simulink model "PTTransmCU"  (R2022b)
settings: Solver=ode45  StartTime=0.0  StopTime=inf  RelTol=1e-3  EnableMultiTasking=on
libraries: simulink x2, CarMaker4SL x1
(part 3 of 5)

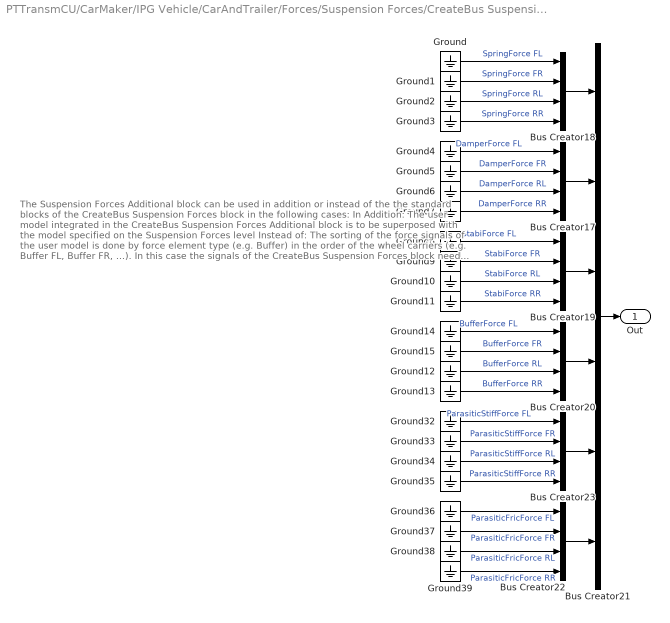
== system PTTransmCU/CarMaker/IPG Vehicle/CarAndTrailer/Forces/Suspension Forces/CreateBus Suspension Forces Additional ==
  note: The Suspension Forces Additional block can be used in addition or instead of the
      | the standard blocks of the CreateBus Suspension Forces block in the following cases:
      |
      | In Addition: The user model integrated in the CreateBus Suspension Forces Additional block is to be superposed with the model specified on the Suspension Forces level
      | Instead of: The sorting of the force signals of the user model is done by force element type (e.g. Buffer) in the order of the wheel carriers (e.g. Buffer FL, Buffer FR, ...). In this case the signals of the CreateBus Suspension Forces block need to be disabled e.g. by manually connecting them to ground signals.
      |
      | ATTENTION : The forces given in the CreateBus Suspension Forces Additional block are internally added to the forces of the Suspension Forces block. If this is not desired, make sure to include a force model only in one of the two levels.
  Bus Creator{17..20,22..23} (6 alike) : BusCreator  Inputs=4
  Bus Creator21 : BusCreator  Inputs=6
  Ground{,1..15,32..39} (24 alike) : Ground
  Out : Outport
  wires:
  Ground1/1 -> Bus Creator18/2  "SpringForce FR"
  Ground9/1 -> Bus Creator19/2  "StabiForce FR"
  Ground8/1 -> Bus Creator19/1  "StabiForce FL"
  Bus Creator22/1 -> Bus Creator21/6
  Bus Creator21/1 -> Out/1
  Ground/1 -> Bus Creator18/1  "SpringForce FL"
  Ground36/1 -> Bus Creator22/1  "ParasiticFricForce FL"
  Ground2/1 -> Bus Creator18/3  "SpringForce RL"
  Ground5/1 -> Bus Creator17/2  "DamperForce FR"
  Ground15/1 -> Bus Creator20/2  "BufferForce FR"
  Ground35/1 -> Bus Creator23/4  "ParasiticStiffForce RR"
  Bus Creator20/1 -> Bus Creator21/4
  Bus Creator17/1 -> Bus Creator21/2
  Ground37/1 -> Bus Creator22/2  "ParasiticFricForce FR"
  Ground4/1 -> Bus Creator17/1  "DamperForce FL"
  Ground33/1 -> Bus Creator23/2  "ParasiticStiffForce FR"
  Bus Creator23/1 -> Bus Creator21/5
  Ground11/1 -> Bus Creator19/4  "StabiForce RR"
  Ground10/1 -> Bus Creator19/3  "StabiForce RL"
  Ground6/1 -> Bus Creator17/3  "DamperForce RL"
  Bus Creator19/1 -> Bus Creator21/3
  Ground7/1 -> Bus Creator17/4  "DamperForce RR"
  Bus Creator18/1 -> Bus Creator21/1
  Ground34/1 -> Bus Creator23/3  "ParasiticStiffForce RL"
  Ground3/1 -> Bus Creator18/4  "SpringForce RR"
  Ground12/1 -> Bus Creator20/3  "BufferForce RL"
  Ground38/1 -> Bus Creator22/3  "ParasiticFricForce RL"
  Ground14/1 -> Bus Creator20/1  "BufferForce FL"
  Ground39/1 -> Bus Creator22/4  "ParasiticFricForce RR"
  Ground32/1 -> Bus Creator23/1  "ParasiticStiffForce FL"
  Ground13/1 -> Bus Creator20/4  "BufferForce RR"

== system PTTransmCU/CarMaker/IPG Vehicle/CarAndTrailer/Forces/Suspension Forces/CreateBus Suspension Forces CtrlOut ==
  note: <Your model here>
  In : Inport
  Bus Creator{,1..3,9} (5 alike) : BusCreator  Inputs=4
  Demux{,2..5} (5 alike) : Demux
  Out : Outport
  wires:
  Bus Creator3/1 -> Bus Creator9/4
  Demux2/4 -> Bus Creator/4  "FL BufferCtrlOut"
  Demux/4 -> Demux5/1  "RR"
  Bus Creator2/1 -> Bus Creator9/3
  Demux3/1 -> Bus Creator1/1  "FR SpringCtrlOut"
  Bus Creator/1 -> Bus Creator9/1
  Demux5/1 -> Bus Creator3/1  "RR SpringCtrlOut"
  Demux5/2 -> Bus Creator3/2  "RR DamperCtrlOut"
  Demux4/2 -> Bus Creator2/2  "RL DamperCtrlOut"
  Demux4/3 -> Bus Creator2/3  "RL StabiCtrlOut"
  Demux2/2 -> Bus Creator/2  "FL DamperCtrlOut"
  Demux/3 -> Demux4/1  "RL"
  Demux5/4 -> Bus Creator3/4  "RR BufferCtrlOut"
  In/1 -> Demux/1
  Demux2/1 -> Bus Creator/1  "FL SpringCtrlOut"
  Demux3/3 -> Bus Creator1/3  "FR StabiCtrlOut"
  Demux3/2 -> Bus Creator1/2  "FR DamperCtrlOut"
  Demux4/1 -> Bus Creator2/1  "RL SpringCtrlOut"
  Demux4/4 -> Bus Creator2/4  "RL BufferCtrlOut"
  Demux2/3 -> Bus Creator/3  "FL StabiCtrlOut"
  Bus Creator1/1 -> Bus Creator9/2
  Bus Creator9/1 -> Out/1
  Demux/1 -> Demux2/1  "FL"
  Demux/2 -> Demux3/1  "FR"
  Demux5/3 -> Bus Creator3/3  "RR StabiCtrlOut"
  Demux3/4 -> Bus Creator1/4  "FR BufferCtrlOut"

== system PTTransmCU/CarMaker/IPG Vehicle/CarAndTrailer/Forces/Suspension Forces/Damper CreateBus CtrlOutOpt ==
  note: <Your model here>
  In : Inport
  Bus Creator{,1..3,9} (5 alike) : BusCreator  Inputs=4
  Demux{,2..5} (5 alike) : Demux
  Out : Outport
  wires:
  Bus Creator/1 -> Bus Creator9/1
  Demux/4 -> Demux5/1  "RR"
  Bus Creator2/1 -> Bus Creator9/3
  Demux5/1 -> Bus Creator3/1  "RR CtrlOutOpt0"
  Bus Creator3/1 -> Bus Creator9/4
  Demux2/4 -> Bus Creator/4  "FL CtrlOutOpt3"
  Demux5/3 -> Bus Creator3/3  "RR CtrlOutOpt2"
  Demux4/3 -> Bus Creator2/3  "RL CtrlOutOpt2"
  Bus Creator1/1 -> Bus Creator9/2
  Demux4/2 -> Bus Creator2/2  "RL CtrlOutOpt1"
  Demux2/2 -> Bus Creator/2  "FL CtrlOutOpt1"
  Demux/2 -> Demux3/1  "FR"
  Demux3/4 -> Bus Creator1/4  "FR CtrlOutOpt3"
  Demux3/1 -> Bus Creator1/1  "FR CtrlOutOpt0"
  Demux4/4 -> Bus Creator2/4  "RL CtrlOutOpt3"
  Demux2/3 -> Bus Creator/3  "FL CtrlOutOpt2"
  Demux3/2 -> Bus Creator1/2  "FR CtrlOutOpt1"
  Demux2/1 -> Bus Creator/1  "FL CtrlOutOpt0"
  Demux3/3 -> Bus Creator1/3  "FR CtrlOutOpt2"
  In/1 -> Demux/1
  Demux5/4 -> Bus Creator3/4  "RR CtrlOutOpt3"
  Demux/3 -> Demux4/1  "RL"
  Bus Creator9/1 -> Out/1
  Demux5/2 -> Bus Creator3/2  "RR CtrlOutOpt1"
  Demux4/1 -> Bus Creator2/1  "RL CtrlOutOpt0"
  Demux/1 -> Demux2/1  "FL"

== system PTTransmCU/CarMaker/IPG Vehicle/CarAndTrailer/Forces/Suspension Forces/FrcSystem CreateBus CtrlOutOpt ==
  note: <Your model here>
  In : Inport
  Bus Creator9 : BusCreator  Inputs=64
  Demux : Demux  Outputs=64
  Out : Outport
  wires:
  In/1 -> Demux/1
  Bus Creator9/1 -> Out/1
  Demux/64 -> Bus Creator9/64  "CtrlOutOpt63"
  Demux/1 -> Bus Creator9/1  "CtrlOutOpt0"
  Demux/2 -> Bus Creator9/2  "CtrlOutOpt1"
  Demux/3 -> Bus Creator9/3  "CtrlOutOpt2"
  Demux/4 -> Bus Creator9/4  "CtrlOutOpt3"
  Demux/5 -> Bus Creator9/5  "CtrlOutOpt4"
  Demux/6 -> Bus Creator9/6  "CtrlOutOpt5"
  Demux/7 -> Bus Creator9/7  "CtrlOutOpt6"
  Demux/8 -> Bus Creator9/8  "CtrlOutOpt7"
  Demux/9 -> Bus Creator9/9  "CtrlOutOpt8"
  Demux/10 -> Bus Creator9/10  "CtrlOutOpt9"
  Demux/11 -> Bus Creator9/11  "CtrlOutOpt10"
  Demux/12 -> Bus Creator9/12  "CtrlOutOpt11"
  Demux/13 -> Bus Creator9/13  "CtrlOutOpt12"
  Demux/14 -> Bus Creator9/14  "CtrlOutOpt13"
  Demux/15 -> Bus Creator9/15  "CtrlOutOpt14"
  Demux/16 -> Bus Creator9/16  "CtrlOutOpt15"
  Demux/17 -> Bus Creator9/17  "CtrlOutOpt16"
  Demux/18 -> Bus Creator9/18  "CtrlOutOpt17"
  Demux/19 -> Bus Creator9/19  "CtrlOutOpt18"
  Demux/20 -> Bus Creator9/20  "CtrlOutOpt19"
  Demux/21 -> Bus Creator9/21  "CtrlOutOpt20"
  Demux/22 -> Bus Creator9/22  "CtrlOutOpt21"
  Demux/23 -> Bus Creator9/23  "CtrlOutOpt22"
  Demux/24 -> Bus Creator9/24  "CtrlOutOpt23"
  Demux/25 -> Bus Creator9/25  "CtrlOutOpt24"
  Demux/26 -> Bus Creator9/26  "CtrlOutOpt25"
  Demux/27 -> Bus Creator9/27  "CtrlOutOpt26"
  Demux/28 -> Bus Creator9/28  "CtrlOutOpt27"
  Demux/29 -> Bus Creator9/29  "CtrlOutOpt28"
  Demux/30 -> Bus Creator9/30  "CtrlOutOpt29"
  Demux/31 -> Bus Creator9/31  "CtrlOutOpt30"
  Demux/32 -> Bus Creator9/32  "CtrlOutOpt31"
  Demux/33 -> Bus Creator9/33  "CtrlOutOpt32"
  Demux/34 -> Bus Creator9/34  "CtrlOutOpt33"
  Demux/35 -> Bus Creator9/35  "CtrlOutOpt34"
  Demux/36 -> Bus Creator9/36  "CtrlOutOpt35"
  Demux/37 -> Bus Creator9/37  "CtrlOutOpt36"
  Demux/38 -> Bus Creator9/38  "CtrlOutOpt37"
  Demux/39 -> Bus Creator9/39  "CtrlOutOpt38"
  Demux/40 -> Bus Creator9/40  "CtrlOutOpt39"
  Demux/41 -> Bus Creator9/41  "CtrlOutOpt40"
  Demux/42 -> Bus Creator9/42  "CtrlOutOpt41"
  Demux/43 -> Bus Creator9/43  "CtrlOutOpt42"
  Demux/44 -> Bus Creator9/44  "CtrlOutOpt43"
  Demux/45 -> Bus Creator9/45  "CtrlOutOpt44"
  Demux/46 -> Bus Creator9/46  "CtrlOutOpt45"
  Demux/47 -> Bus Creator9/47  "CtrlOutOpt46"
  Demux/48 -> Bus Creator9/48  "CtrlOutOpt47"
  Demux/49 -> Bus Creator9/49  "CtrlOutOpt48"
  Demux/50 -> Bus Creator9/50  "CtrlOutOpt49"
  Demux/51 -> Bus Creator9/51  "CtrlOutOpt50"
  Demux/52 -> Bus Creator9/52  "CtrlOutOpt51"
  Demux/53 -> Bus Creator9/53  "CtrlOutOpt52"
  Demux/54 -> Bus Creator9/54  "CtrlOutOpt53"
  Demux/55 -> Bus Creator9/55  "CtrlOutOpt54"
  Demux/56 -> Bus Creator9/56  "CtrlOutOpt55"
  Demux/57 -> Bus Creator9/57  "CtrlOutOpt56"
  Demux/58 -> Bus Creator9/58  "CtrlOutOpt57"
  Demux/59 -> Bus Creator9/59  "CtrlOutOpt58"
  Demux/60 -> Bus Creator9/60  "CtrlOutOpt59"
  Demux/61 -> Bus Creator9/61  "CtrlOutOpt60"
  Demux/62 -> Bus Creator9/62  "CtrlOutOpt61"
  Demux/63 -> Bus Creator9/63  "CtrlOutOpt62"

== system PTTransmCU/CarMaker/IPG Vehicle/CarAndTrailer/Forces/Suspension Forces/Spring CreateBus CtrlOutOpt ==
  note: <Your model here>
  In : Inport
  Bus Creator{,1..3,9} (5 alike) : BusCreator  Inputs=4
  Demux{,2..5} (5 alike) : Demux
  Out : Outport
  wires:
  Bus Creator/1 -> Bus Creator9/1
  Demux/4 -> Demux5/1  "RR"
  Bus Creator2/1 -> Bus Creator9/3
  Demux5/1 -> Bus Creator3/1  "RR CtrlOutOpt0"
  Bus Creator3/1 -> Bus Creator9/4
  Demux2/4 -> Bus Creator/4  "FL CtrlOutOpt3"
  Demux5/3 -> Bus Creator3/3  "RR CtrlOutOpt2"
  Demux4/3 -> Bus Creator2/3  "RL CtrlOutOpt2"
  Bus Creator1/1 -> Bus Creator9/2
  Demux4/2 -> Bus Creator2/2  "RL CtrlOutOpt1"
  Demux2/2 -> Bus Creator/2  "FL CtrlOutOpt1"
  Demux/2 -> Demux3/1  "FR"
  Demux3/4 -> Bus Creator1/4  "FR CtrlOutOpt3"
  Demux3/1 -> Bus Creator1/1  "FR CtrlOutOpt0"
  Demux4/4 -> Bus Creator2/4  "RL CtrlOutOpt3"
  Demux2/3 -> Bus Creator/3  "FL CtrlOutOpt2"
  Demux3/2 -> Bus Creator1/2  "FR CtrlOutOpt1"
  Demux2/1 -> Bus Creator/1  "FL CtrlOutOpt0"
  Demux3/3 -> Bus Creator1/3  "FR CtrlOutOpt2"
  In/1 -> Demux/1
  Demux5/4 -> Bus Creator3/4  "RR CtrlOutOpt3"
  Demux/3 -> Demux4/1  "RL"
  Bus Creator9/1 -> Out/1
  Demux5/2 -> Bus Creator3/2  "RR CtrlOutOpt1"
  Demux4/1 -> Bus Creator2/1  "RL CtrlOutOpt0"
  Demux/1 -> Demux2/1  "FL"

== system PTTransmCU/CarMaker/IPG Vehicle/CarAndTrailer/Forces/Suspension Forces/Stabi CreateBus CtrlOutOpt ==
  note: <Your model here>
  In : Inport
  Bus Creator{,1..3,9} (5 alike) : BusCreator  Inputs=4
  Demux{,2..5} (5 alike) : Demux
  Out : Outport
  wires:
  Bus Creator/1 -> Bus Creator9/1
  Demux/4 -> Demux5/1  "RR"
  Bus Creator2/1 -> Bus Creator9/3
  Demux5/1 -> Bus Creator3/1  "RR CtrlOutOpt0"
  Bus Creator3/1 -> Bus Creator9/4
  Demux2/4 -> Bus Creator/4  "FL CtrlOutOpt3"
  Demux5/3 -> Bus Creator3/3  "RR CtrlOutOpt2"
  Demux4/3 -> Bus Creator2/3  "RL CtrlOutOpt2"
  Bus Creator1/1 -> Bus Creator9/2
  Demux4/2 -> Bus Creator2/2  "RL CtrlOutOpt1"
  Demux2/2 -> Bus Creator/2  "FL CtrlOutOpt1"
  Demux/2 -> Demux3/1  "FR"
  Demux3/4 -> Bus Creator1/4  "FR CtrlOutOpt3"
  Demux3/1 -> Bus Creator1/1  "FR CtrlOutOpt0"
  Demux4/4 -> Bus Creator2/4  "RL CtrlOutOpt3"
  Demux2/3 -> Bus Creator/3  "FL CtrlOutOpt2"
  Demux3/2 -> Bus Creator1/2  "FR CtrlOutOpt1"
  Demux2/1 -> Bus Creator/1  "FL CtrlOutOpt0"
  Demux3/3 -> Bus Creator1/3  "FR CtrlOutOpt2"
  In/1 -> Demux/1
  Demux5/4 -> Bus Creator3/4  "RR CtrlOutOpt3"
  Demux/3 -> Demux4/1  "RL"
  Bus Creator9/1 -> Out/1
  Demux5/2 -> Bus Creator3/2  "RR CtrlOutOpt1"
  Demux4/1 -> Bus Creator2/1  "RL CtrlOutOpt0"
  Demux/1 -> Demux2/1  "FL"

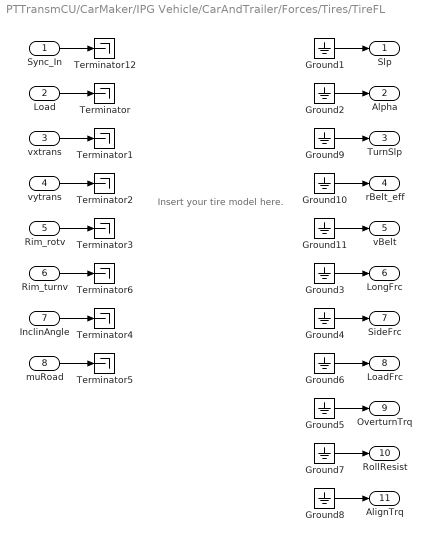
== system PTTransmCU/CarMaker/IPG Vehicle/CarAndTrailer/Forces/Tires/TireFL ==
  note: Insert your tire model here.
  Sync_In : Inport
  Load : Inport  Port=2
  vxtrans : Inport  Port=3
  vytrans : Inport  Port=4
  Rim_rotv : Inport  Port=5
  Rim_turnv : Inport  Port=6
  InclinAngle : Inport  Port=7
  muRoad : Inport  Port=8
  Ground{1..11} (11 alike) : Ground
  Terminator{,1..6,12} (8 alike) : Terminator
  Slp : Outport  VectorParamsAs1DForOutWhenUnconnected=off
  Alpha : Outport  Port=2  VectorParamsAs1DForOutWhenUnconnected=off
  TurnSlp : Outport  Port=3  VectorParamsAs1DForOutWhenUnconnected=off
  rBelt_eff : Outport  Port=4  VectorParamsAs1DForOutWhenUnconnected=off
  vBelt : Outport  Port=5  VectorParamsAs1DForOutWhenUnconnected=off
  LongFrc : Outport  Port=6  VectorParamsAs1DForOutWhenUnconnected=off
  SideFrc : Outport  Port=7  VectorParamsAs1DForOutWhenUnconnected=off
  LoadFrc : Outport  Port=8  VectorParamsAs1DForOutWhenUnconnected=off
  OverturnTrq : Outport  Port=9  VectorParamsAs1DForOutWhenUnconnected=off
  RollResist : Outport  Port=10  VectorParamsAs1DForOutWhenUnconnected=off
  AlignTrq : Outport  Port=11  VectorParamsAs1DForOutWhenUnconnected=off
  wires:
  Ground11/1 -> vBelt/1
  Ground10/1 -> rBelt_eff/1
  Ground9/1 -> TurnSlp/1
  Rim_turnv/1 -> Terminator6/1
  Sync_In/1 -> Terminator12/1
  Ground2/1 -> Alpha/1
  Ground3/1 -> LongFrc/1
  Ground4/1 -> SideFrc/1
  Ground5/1 -> OverturnTrq/1
  vxtrans/1 -> Terminator1/1
  vytrans/1 -> Terminator2/1
  Rim_rotv/1 -> Terminator3/1
  InclinAngle/1 -> Terminator4/1
  muRoad/1 -> Terminator5/1
  Load/1 -> Terminator/1
  Ground1/1 -> Slp/1
  Ground6/1 -> LoadFrc/1
  Ground7/1 -> RollResist/1
  Ground8/1 -> AlignTrq/1

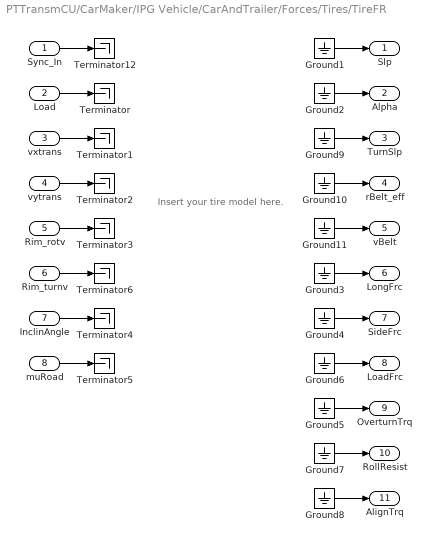
== system PTTransmCU/CarMaker/IPG Vehicle/CarAndTrailer/Forces/Tires/TireFR ==
  note: Insert your tire model here.
  Sync_In : Inport
  Load : Inport  Port=2
  vxtrans : Inport  Port=3
  vytrans : Inport  Port=4
  Rim_rotv : Inport  Port=5
  Rim_turnv : Inport  Port=6
  InclinAngle : Inport  Port=7
  muRoad : Inport  Port=8
  Ground{1..11} (11 alike) : Ground
  Terminator{,1..6,12} (8 alike) : Terminator
  Slp : Outport  VectorParamsAs1DForOutWhenUnconnected=off
  Alpha : Outport  Port=2  VectorParamsAs1DForOutWhenUnconnected=off
  TurnSlp : Outport  Port=3  VectorParamsAs1DForOutWhenUnconnected=off
  rBelt_eff : Outport  Port=4  VectorParamsAs1DForOutWhenUnconnected=off
  vBelt : Outport  Port=5  VectorParamsAs1DForOutWhenUnconnected=off
  LongFrc : Outport  Port=6  VectorParamsAs1DForOutWhenUnconnected=off
  SideFrc : Outport  Port=7  VectorParamsAs1DForOutWhenUnconnected=off
  LoadFrc : Outport  Port=8  VectorParamsAs1DForOutWhenUnconnected=off
  OverturnTrq : Outport  Port=9  VectorParamsAs1DForOutWhenUnconnected=off
  RollResist : Outport  Port=10  VectorParamsAs1DForOutWhenUnconnected=off
  AlignTrq : Outport  Port=11  VectorParamsAs1DForOutWhenUnconnected=off
  wires:
  Ground11/1 -> vBelt/1
  Ground10/1 -> rBelt_eff/1
  Ground9/1 -> TurnSlp/1
  Rim_turnv/1 -> Terminator6/1
  Sync_In/1 -> Terminator12/1
  Ground2/1 -> Alpha/1
  Ground3/1 -> LongFrc/1
  Ground4/1 -> SideFrc/1
  Ground5/1 -> OverturnTrq/1
  vxtrans/1 -> Terminator1/1
  vytrans/1 -> Terminator2/1
  Rim_rotv/1 -> Terminator3/1
  InclinAngle/1 -> Terminator4/1
  muRoad/1 -> Terminator5/1
  Load/1 -> Terminator/1
  Ground1/1 -> Slp/1
  Ground6/1 -> LoadFrc/1
  Ground7/1 -> RollResist/1
  Ground8/1 -> AlignTrq/1

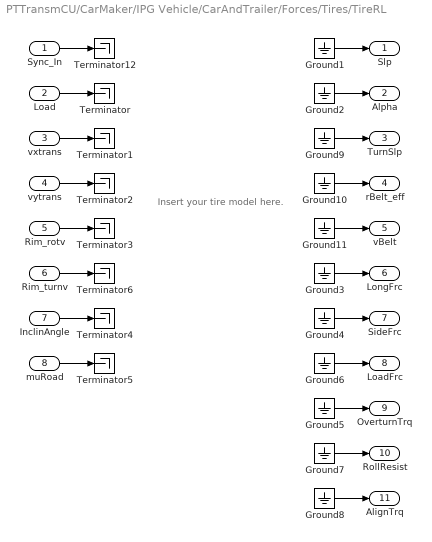
== system PTTransmCU/CarMaker/IPG Vehicle/CarAndTrailer/Forces/Tires/TireRL ==
  note: Insert your tire model here.
  Sync_In : Inport
  Load : Inport  Port=2
  vxtrans : Inport  Port=3
  vytrans : Inport  Port=4
  Rim_rotv : Inport  Port=5
  Rim_turnv : Inport  Port=6
  InclinAngle : Inport  Port=7
  muRoad : Inport  Port=8
  Ground{1..11} (11 alike) : Ground
  Terminator{,1..6,12} (8 alike) : Terminator
  Slp : Outport  VectorParamsAs1DForOutWhenUnconnected=off
  Alpha : Outport  Port=2  VectorParamsAs1DForOutWhenUnconnected=off
  TurnSlp : Outport  Port=3  VectorParamsAs1DForOutWhenUnconnected=off
  rBelt_eff : Outport  Port=4  VectorParamsAs1DForOutWhenUnconnected=off
  vBelt : Outport  Port=5  VectorParamsAs1DForOutWhenUnconnected=off
  LongFrc : Outport  Port=6  VectorParamsAs1DForOutWhenUnconnected=off
  SideFrc : Outport  Port=7  VectorParamsAs1DForOutWhenUnconnected=off
  LoadFrc : Outport  Port=8  VectorParamsAs1DForOutWhenUnconnected=off
  OverturnTrq : Outport  Port=9  VectorParamsAs1DForOutWhenUnconnected=off
  RollResist : Outport  Port=10  VectorParamsAs1DForOutWhenUnconnected=off
  AlignTrq : Outport  Port=11  VectorParamsAs1DForOutWhenUnconnected=off
  wires:
  Ground11/1 -> vBelt/1
  Ground10/1 -> rBelt_eff/1
  Ground9/1 -> TurnSlp/1
  Rim_turnv/1 -> Terminator6/1
  Sync_In/1 -> Terminator12/1
  Ground2/1 -> Alpha/1
  Ground3/1 -> LongFrc/1
  Ground4/1 -> SideFrc/1
  Ground5/1 -> OverturnTrq/1
  vxtrans/1 -> Terminator1/1
  vytrans/1 -> Terminator2/1
  Rim_rotv/1 -> Terminator3/1
  InclinAngle/1 -> Terminator4/1
  muRoad/1 -> Terminator5/1
  Load/1 -> Terminator/1
  Ground1/1 -> Slp/1
  Ground6/1 -> LoadFrc/1
  Ground7/1 -> RollResist/1
  Ground8/1 -> AlignTrq/1

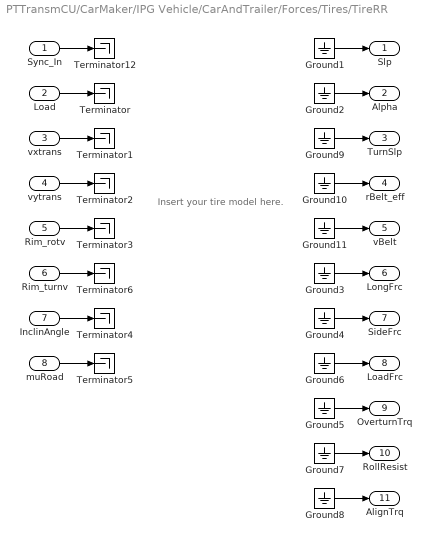
== system PTTransmCU/CarMaker/IPG Vehicle/CarAndTrailer/Forces/Tires/TireRR ==
  note: Insert your tire model here.
  Sync_In : Inport
  Load : Inport  Port=2
  vxtrans : Inport  Port=3
  vytrans : Inport  Port=4
  Rim_rotv : Inport  Port=5
  Rim_turnv : Inport  Port=6
  InclinAngle : Inport  Port=7
  muRoad : Inport  Port=8
  Ground{1..11} (11 alike) : Ground
  Terminator{,1..6,12} (8 alike) : Terminator
  Slp : Outport  VectorParamsAs1DForOutWhenUnconnected=off
  Alpha : Outport  Port=2  VectorParamsAs1DForOutWhenUnconnected=off
  TurnSlp : Outport  Port=3  VectorParamsAs1DForOutWhenUnconnected=off
  rBelt_eff : Outport  Port=4  VectorParamsAs1DForOutWhenUnconnected=off
  vBelt : Outport  Port=5  VectorParamsAs1DForOutWhenUnconnected=off
  LongFrc : Outport  Port=6  VectorParamsAs1DForOutWhenUnconnected=off
  SideFrc : Outport  Port=7  VectorParamsAs1DForOutWhenUnconnected=off
  LoadFrc : Outport  Port=8  VectorParamsAs1DForOutWhenUnconnected=off
  OverturnTrq : Outport  Port=9  VectorParamsAs1DForOutWhenUnconnected=off
  RollResist : Outport  Port=10  VectorParamsAs1DForOutWhenUnconnected=off
  AlignTrq : Outport  Port=11  VectorParamsAs1DForOutWhenUnconnected=off
  wires:
  Ground11/1 -> vBelt/1
  Ground10/1 -> rBelt_eff/1
  Ground9/1 -> TurnSlp/1
  Rim_turnv/1 -> Terminator6/1
  Sync_In/1 -> Terminator12/1
  Ground2/1 -> Alpha/1
  Ground3/1 -> LongFrc/1
  Ground4/1 -> SideFrc/1
  Ground5/1 -> OverturnTrq/1
  vxtrans/1 -> Terminator1/1
  vytrans/1 -> Terminator2/1
  Rim_rotv/1 -> Terminator3/1
  InclinAngle/1 -> Terminator4/1
  muRoad/1 -> Terminator5/1
  Load/1 -> Terminator/1
  Ground1/1 -> Slp/1
  Ground6/1 -> LoadFrc/1
  Ground7/1 -> RollResist/1
  Ground8/1 -> AlignTrq/1

== system PTTransmCU/CarMaker/IPG Vehicle/PowerTrain/TCU Example/PTTransmCU_In/CreateBus TCU ClutchIn0 ==
  In : Inport
  BusCreator : BusCreator  Inputs=7
  Demux : Demux  Outputs=7
      settings: DisplayOption=none
  Out : Outport  VectorParamsAs1DForOutWhenUnconnected=off
  wires:
  Demux/7 -> BusCreator/7  "TCU ClutchIn0 i_TrqIn2Out"
  Demux/6 -> BusCreator/6  "TCU ClutchIn0 Trq_out_trg"
  Demux/5 -> BusCreator/5  "TCU ClutchIn0 Trq_out"
  Demux/4 -> BusCreator/4  "TCU ClutchIn0 Trq_in"
  Demux/3 -> BusCreator/3  "TCU ClutchIn0 rotv_out_trg"
  Demux/2 -> BusCreator/2  "TCU ClutchIn0 rotv_out"
  Demux/1 -> BusCreator/1  "TCU ClutchIn0 rotv_in"
  BusCreator/1 -> Out/1
  In/1 -> Demux/1

== system PTTransmCU/CarMaker/IPG Vehicle/PowerTrain/TCU Example/PTTransmCU_In/CreateBus TCU ClutchIn1 ==
  In : Inport
  BusCreator : BusCreator  Inputs=7
  Demux : Demux  Outputs=7
      settings: DisplayOption=none
  Out : Outport  VectorParamsAs1DForOutWhenUnconnected=off
  wires:
  Demux/7 -> BusCreator/7  "TCU ClutchIn1 i_TrqIn2Out"
  Demux/6 -> BusCreator/6  "TCU ClutchIn1 Trq_out_trg"
  Demux/5 -> BusCreator/5  "TCU ClutchIn1 Trq_out"
  Demux/4 -> BusCreator/4  "TCU ClutchIn1 Trq_in"
  Demux/3 -> BusCreator/3  "TCU ClutchIn1 rotv_out_trg"
  Demux/2 -> BusCreator/2  "TCU ClutchIn1 rotv_out"
  Demux/1 -> BusCreator/1  "TCU ClutchIn1 rotv_in"
  BusCreator/1 -> Out/1
  In/1 -> Demux/1

== system PTTransmCU/CarMaker/IPG Vehicle/PowerTrain/TCU Example/PTTransmCU_In/CreateBus TCU ClutchIn10 ==
  In : Inport
  BusCreator : BusCreator  Inputs=7
  Demux : Demux  Outputs=7
      settings: DisplayOption=none
  Out : Outport  VectorParamsAs1DForOutWhenUnconnected=off
  wires:
  Demux/7 -> BusCreator/7  "TCU ClutchIn10 i_TrqIn2Out"
  Demux/6 -> BusCreator/6  "TCU ClutchIn10 Trq_out_trg"
  Demux/5 -> BusCreator/5  "TCU ClutchIn10 Trq_out"
  Demux/4 -> BusCreator/4  "TCU ClutchIn10 Trq_in"
  Demux/3 -> BusCreator/3  "TCU ClutchIn10 rotv_out_trg"
  Demux/2 -> BusCreator/2  "TCU ClutchIn10 rotv_out"
  Demux/1 -> BusCreator/1  "TCU ClutchIn10 rotv_in"
  BusCreator/1 -> Out/1
  In/1 -> Demux/1

== system PTTransmCU/CarMaker/IPG Vehicle/PowerTrain/TCU Example/PTTransmCU_In/CreateBus TCU ClutchIn11 ==
  In : Inport
  BusCreator : BusCreator  Inputs=7
  Demux : Demux  Outputs=7
      settings: DisplayOption=none
  Out : Outport  VectorParamsAs1DForOutWhenUnconnected=off
  wires:
  Demux/7 -> BusCreator/7  "TCU ClutchIn10 i_TrqIn2Out"
  Demux/6 -> BusCreator/6  "TCU ClutchIn10 Trq_out_trg"
  Demux/5 -> BusCreator/5  "TCU ClutchIn10 Trq_out"
  Demux/4 -> BusCreator/4  "TCU ClutchIn10 Trq_in"
  Demux/3 -> BusCreator/3  "TCU ClutchIn10 rotv_out_trg"
  Demux/2 -> BusCreator/2  "TCU ClutchIn10 rotv_out"
  Demux/1 -> BusCreator/1  "TCU ClutchIn10 rotv_in"
  BusCreator/1 -> Out/1
  In/1 -> Demux/1

== system PTTransmCU/CarMaker/IPG Vehicle/PowerTrain/TCU Example/PTTransmCU_In/CreateBus TCU ClutchIn2 ==
  In : Inport
  BusCreator : BusCreator  Inputs=7
  Demux : Demux  Outputs=7
      settings: DisplayOption=none
  Out : Outport  VectorParamsAs1DForOutWhenUnconnected=off
  wires:
  Demux/7 -> BusCreator/7  "TCU ClutchIn2 i_TrqIn2Out"
  Demux/6 -> BusCreator/6  "TCU ClutchIn2 Trq_out_trg"
  Demux/5 -> BusCreator/5  "TCU ClutchIn2 Trq_out"
  Demux/4 -> BusCreator/4  "TCU ClutchIn2 Trq_in"
  Demux/3 -> BusCreator/3  "TCU ClutchIn2 rotv_out_trg"
  Demux/2 -> BusCreator/2  "TCU ClutchIn2 rotv_out"
  Demux/1 -> BusCreator/1  "TCU ClutchIn2 rotv_in"
  BusCreator/1 -> Out/1
  In/1 -> Demux/1

== system PTTransmCU/CarMaker/IPG Vehicle/PowerTrain/TCU Example/PTTransmCU_In/CreateBus TCU ClutchIn3 ==
  In : Inport
  BusCreator : BusCreator  Inputs=7
  Demux : Demux  Outputs=7
      settings: DisplayOption=none
  Out : Outport  VectorParamsAs1DForOutWhenUnconnected=off
  wires:
  Demux/7 -> BusCreator/7  "TCU ClutchIn3 i_TrqIn2Out"
  Demux/6 -> BusCreator/6  "TCU ClutchIn3 Trq_out_trg"
  Demux/5 -> BusCreator/5  "TCU ClutchIn3 Trq_out"
  Demux/4 -> BusCreator/4  "TCU ClutchIn3 Trq_in"
  Demux/3 -> BusCreator/3  "TCU ClutchIn3 rotv_out_trg"
  Demux/2 -> BusCreator/2  "TCU ClutchIn3 rotv_out"
  Demux/1 -> BusCreator/1  "TCU ClutchIn3 rotv_in"
  BusCreator/1 -> Out/1
  In/1 -> Demux/1

== system PTTransmCU/CarMaker/IPG Vehicle/PowerTrain/TCU Example/PTTransmCU_In/CreateBus TCU ClutchIn4 ==
  In : Inport
  BusCreator : BusCreator  Inputs=7
  Demux : Demux  Outputs=7
      settings: DisplayOption=none
  Out : Outport  VectorParamsAs1DForOutWhenUnconnected=off
  wires:
  Demux/7 -> BusCreator/7  "TCU ClutchIn4 i_TrqIn2Out"
  Demux/6 -> BusCreator/6  "TCU ClutchIn4 Trq_out_trg"
  Demux/5 -> BusCreator/5  "TCU ClutchIn4 Trq_out"
  Demux/4 -> BusCreator/4  "TCU ClutchIn4 Trq_in"
  Demux/3 -> BusCreator/3  "TCU ClutchIn4 rotv_out_trg"
  Demux/2 -> BusCreator/2  "TCU ClutchIn4 rotv_out"
  Demux/1 -> BusCreator/1  "TCU ClutchIn4 rotv_in"
  BusCreator/1 -> Out/1
  In/1 -> Demux/1

== system PTTransmCU/CarMaker/IPG Vehicle/PowerTrain/TCU Example/PTTransmCU_In/CreateBus TCU ClutchIn5 ==
  In : Inport
  BusCreator : BusCreator  Inputs=7
  Demux : Demux  Outputs=7
      settings: DisplayOption=none
  Out : Outport  VectorParamsAs1DForOutWhenUnconnected=off
  wires:
  Demux/7 -> BusCreator/7  "TCU ClutchIn5 i_TrqIn2Out"
  Demux/6 -> BusCreator/6  "TCU ClutchIn5 Trq_out_trg"
  Demux/5 -> BusCreator/5  "TCU ClutchIn5 Trq_out"
  Demux/4 -> BusCreator/4  "TCU ClutchIn5 Trq_in"
  Demux/3 -> BusCreator/3  "TCU ClutchIn5 rotv_out_trg"
  Demux/2 -> BusCreator/2  "TCU ClutchIn5 rotv_out"
  Demux/1 -> BusCreator/1  "TCU ClutchIn5 rotv_in"
  BusCreator/1 -> Out/1
  In/1 -> Demux/1

== system PTTransmCU/CarMaker/IPG Vehicle/PowerTrain/TCU Example/PTTransmCU_In/CreateBus TCU ClutchIn6 ==
  In : Inport
  BusCreator : BusCreator  Inputs=7
  Demux : Demux  Outputs=7
      settings: DisplayOption=none
  Out : Outport  VectorParamsAs1DForOutWhenUnconnected=off
  wires:
  Demux/7 -> BusCreator/7  "TCU ClutchIn6 i_TrqIn2Out"
  Demux/6 -> BusCreator/6  "TCU ClutchIn6 Trq_out_trg"
  Demux/5 -> BusCreator/5  "TCU ClutchIn6 Trq_out"
  Demux/4 -> BusCreator/4  "TCU ClutchIn6 Trq_in"
  Demux/3 -> BusCreator/3  "TCU ClutchIn6 rotv_out_trg"
  Demux/2 -> BusCreator/2  "TCU ClutchIn6 rotv_out"
  Demux/1 -> BusCreator/1  "TCU ClutchIn6 rotv_in"
  BusCreator/1 -> Out/1
  In/1 -> Demux/1

== system PTTransmCU/CarMaker/IPG Vehicle/PowerTrain/TCU Example/PTTransmCU_In/CreateBus TCU ClutchIn7 ==
  In : Inport
  BusCreator : BusCreator  Inputs=7
  Demux : Demux  Outputs=7
      settings: DisplayOption=none
  Out : Outport  VectorParamsAs1DForOutWhenUnconnected=off
  wires:
  Demux/7 -> BusCreator/7  "TCU ClutchIn7 i_TrqIn2Out"
  Demux/6 -> BusCreator/6  "TCU ClutchIn7 Trq_out_trg"
  Demux/5 -> BusCreator/5  "TCU ClutchIn7 Trq_out"
  Demux/4 -> BusCreator/4  "TCU ClutchIn7 Trq_in"
  Demux/3 -> BusCreator/3  "TCU ClutchIn7 rotv_out_trg"
  Demux/2 -> BusCreator/2  "TCU ClutchIn7 rotv_out"
  Demux/1 -> BusCreator/1  "TCU ClutchIn7 rotv_in"
  BusCreator/1 -> Out/1
  In/1 -> Demux/1

== system PTTransmCU/CarMaker/IPG Vehicle/PowerTrain/TCU Example/PTTransmCU_In/CreateBus TCU ClutchIn8 ==
  In : Inport
  BusCreator : BusCreator  Inputs=7
  Demux : Demux  Outputs=7
      settings: DisplayOption=none
  Out : Outport  VectorParamsAs1DForOutWhenUnconnected=off
  wires:
  Demux/7 -> BusCreator/7  "TCU ClutchIn8 i_TrqIn2Out"
  Demux/6 -> BusCreator/6  "TCU ClutchIn8 Trq_out_trg"
  Demux/5 -> BusCreator/5  "TCU ClutchIn8 Trq_out"
  Demux/4 -> BusCreator/4  "TCU ClutchIn8 Trq_in"
  Demux/3 -> BusCreator/3  "TCU ClutchIn8 rotv_out_trg"
  Demux/2 -> BusCreator/2  "TCU ClutchIn8 rotv_out"
  Demux/1 -> BusCreator/1  "TCU ClutchIn8 rotv_in"
  BusCreator/1 -> Out/1
  In/1 -> Demux/1

== system PTTransmCU/CarMaker/IPG Vehicle/PowerTrain/TCU Example/PTTransmCU_In/CreateBus TCU ClutchIn9 ==
  In : Inport
  BusCreator : BusCreator  Inputs=7
  Demux : Demux  Outputs=7
      settings: DisplayOption=none
  Out : Outport  VectorParamsAs1DForOutWhenUnconnected=off
  wires:
  Demux/7 -> BusCreator/7  "TCU ClutchIn9 i_TrqIn2Out"
  Demux/6 -> BusCreator/6  "TCU ClutchIn9 Trq_out_trg"
  Demux/5 -> BusCreator/5  "TCU ClutchIn9 Trq_out"
  Demux/4 -> BusCreator/4  "TCU ClutchIn9 Trq_in"
  Demux/3 -> BusCreator/3  "TCU ClutchIn9 rotv_out_trg"
  Demux/2 -> BusCreator/2  "TCU ClutchIn9 rotv_out"
  Demux/1 -> BusCreator/1  "TCU ClutchIn9 rotv_in"
  BusCreator/1 -> Out/1
  In/1 -> Demux/1

== system PTTransmCU/CarMaker/IPG Vehicle/PowerTrain/TCU Example/PTTransmCU_In/CreateBus TCU ClutchOut0 ==
  In : Inport
  BusCreator : BusCreator  Inputs=1
  Demux : Demux  Outputs=1
      settings: DisplayOption=none
  Out : Outport  VectorParamsAs1DForOutWhenUnconnected=off
  wires:
  Demux/1 -> BusCreator/1  "TCU ClutchOut0 Pos"
  BusCreator/1 -> Out/1
  In/1 -> Demux/1

== system PTTransmCU/CarMaker/IPG Vehicle/PowerTrain/TCU Example/PTTransmCU_In/CreateBus TCU ClutchOut1 ==
  In : Inport
  BusCreator : BusCreator  Inputs=1
  Demux : Demux  Outputs=1
      settings: DisplayOption=none
  Out : Outport  VectorParamsAs1DForOutWhenUnconnected=off
  wires:
  Demux/1 -> BusCreator/1  "TCU ClutchOut1 Pos"
  BusCreator/1 -> Out/1
  In/1 -> Demux/1

== system PTTransmCU/CarMaker/IPG Vehicle/PowerTrain/TCU Example/PTTransmCU_In/CreateBus TCU ClutchOut10 ==
  In : Inport
  BusCreator : BusCreator  Inputs=1
  Demux : Demux  Outputs=1
      settings: DisplayOption=none
  Out : Outport  VectorParamsAs1DForOutWhenUnconnected=off
  wires:
  Demux/1 -> BusCreator/1  "TCU ClutchOut10 Pos"
  BusCreator/1 -> Out/1
  In/1 -> Demux/1

== system PTTransmCU/CarMaker/IPG Vehicle/PowerTrain/TCU Example/PTTransmCU_In/CreateBus TCU ClutchOut11 ==
  In : Inport
  BusCreator : BusCreator  Inputs=1
  Demux : Demux  Outputs=1
      settings: DisplayOption=none
  Out : Outport  VectorParamsAs1DForOutWhenUnconnected=off
  wires:
  Demux/1 -> BusCreator/1  "TCU ClutchOut11 Pos"
  BusCreator/1 -> Out/1
  In/1 -> Demux/1

== system PTTransmCU/CarMaker/IPG Vehicle/PowerTrain/TCU Example/PTTransmCU_In/CreateBus TCU ClutchOut2 ==
  In : Inport
  BusCreator : BusCreator  Inputs=1
  Demux : Demux  Outputs=1
      settings: DisplayOption=none
  Out : Outport  VectorParamsAs1DForOutWhenUnconnected=off
  wires:
  Demux/1 -> BusCreator/1  "TCU ClutchOut2 Pos"
  BusCreator/1 -> Out/1
  In/1 -> Demux/1

== system PTTransmCU/CarMaker/IPG Vehicle/PowerTrain/TCU Example/PTTransmCU_In/CreateBus TCU ClutchOut3 ==
  In : Inport
  BusCreator : BusCreator  Inputs=1
  Demux : Demux  Outputs=1
      settings: DisplayOption=none
  Out : Outport  VectorParamsAs1DForOutWhenUnconnected=off
  wires:
  Demux/1 -> BusCreator/1  "TCU ClutchOut3 Pos"
  BusCreator/1 -> Out/1
  In/1 -> Demux/1

== system PTTransmCU/CarMaker/IPG Vehicle/PowerTrain/TCU Example/PTTransmCU_In/CreateBus TCU ClutchOut4 ==
  In : Inport
  BusCreator : BusCreator  Inputs=1
  Demux : Demux  Outputs=1
      settings: DisplayOption=none
  Out : Outport  VectorParamsAs1DForOutWhenUnconnected=off
  wires:
  Demux/1 -> BusCreator/1  "TCU ClutchOut4 Pos"
  BusCreator/1 -> Out/1
  In/1 -> Demux/1

== system PTTransmCU/CarMaker/IPG Vehicle/PowerTrain/TCU Example/PTTransmCU_In/CreateBus TCU ClutchOut5 ==
  In : Inport
  BusCreator : BusCreator  Inputs=1
  Demux : Demux  Outputs=1
      settings: DisplayOption=none
  Out : Outport  VectorParamsAs1DForOutWhenUnconnected=off
  wires:
  Demux/1 -> BusCreator/1  "TCU ClutchOut5 Pos"
  BusCreator/1 -> Out/1
  In/1 -> Demux/1

== system PTTransmCU/CarMaker/IPG Vehicle/PowerTrain/TCU Example/PTTransmCU_In/CreateBus TCU ClutchOut6 ==
  In : Inport
  BusCreator : BusCreator  Inputs=1
  Demux : Demux  Outputs=1
      settings: DisplayOption=none
  Out : Outport  VectorParamsAs1DForOutWhenUnconnected=off
  wires:
  Demux/1 -> BusCreator/1  "TCU ClutchOut6 Pos"
  BusCreator/1 -> Out/1
  In/1 -> Demux/1

== system PTTransmCU/CarMaker/IPG Vehicle/PowerTrain/TCU Example/PTTransmCU_In/CreateBus TCU ClutchOut7 ==
  In : Inport
  BusCreator : BusCreator  Inputs=1
  Demux : Demux  Outputs=1
      settings: DisplayOption=none
  Out : Outport  VectorParamsAs1DForOutWhenUnconnected=off
  wires:
  Demux/1 -> BusCreator/1  "TCU ClutchOut7 Pos"
  BusCreator/1 -> Out/1
  In/1 -> Demux/1

== system PTTransmCU/CarMaker/IPG Vehicle/PowerTrain/TCU Example/PTTransmCU_In/CreateBus TCU ClutchOut8 ==
  In : Inport
  BusCreator : BusCreator  Inputs=1
  Demux : Demux  Outputs=1
      settings: DisplayOption=none
  Out : Outport  VectorParamsAs1DForOutWhenUnconnected=off
  wires:
  Demux/1 -> BusCreator/1  "TCU ClutchOut8 Pos"
  BusCreator/1 -> Out/1
  In/1 -> Demux/1

== system PTTransmCU/CarMaker/IPG Vehicle/PowerTrain/TCU Example/PTTransmCU_In/CreateBus TCU ClutchOut9 ==
  In : Inport
  BusCreator : BusCreator  Inputs=1
  Demux : Demux  Outputs=1
      settings: DisplayOption=none
  Out : Outport  VectorParamsAs1DForOutWhenUnconnected=off
  wires:
  Demux/1 -> BusCreator/1  "TCU ClutchOut9 Pos"
  BusCreator/1 -> Out/1
  In/1 -> Demux/1

== system PTTransmCU/CarMaker/IPG Vehicle/PowerTrain/TCU Example/PTTransmCU_In/CreateBus TCU GearboxIn0 ==
  In : Inport
  BusCreator : BusCreator  Inputs=23
  Demux : Demux  Outputs=23
      settings: DisplayOption=none
  Out : Outport  VectorParamsAs1DForOutWhenUnconnected=off
  wires:
  Demux/23 -> BusCreator/23  "TCU GearboxIn0 Clutch_dis i_TrqIn2Out"
  Demux/22 -> BusCreator/22  "TCU GearboxIn0 Clutch_dis Trq_out_trg"
  Demux/21 -> BusCreator/21  "TCU GearboxIn0 Clutch_dis Trq_out"
  Demux/20 -> BusCreator/20  "TCU GearboxIn0 Clutch_dis Trq_in"
  Demux/19 -> BusCreator/19  "TCU GearboxIn0 Clutch_dis rotv_out_trg"
  Demux/18 -> BusCreator/18  "TCU GearboxIn0 Clutch_dis rotv_out"
  Demux/17 -> BusCreator/17  "TCU GearboxIn0 Clutch_dis rotv_in"
  Demux/16 -> BusCreator/16  "TCU GearboxIn0 Clutch i_TrqIn2Out"
  Demux/15 -> BusCreator/15  "TCU GearboxIn0 Clutch Trq_out_trg"
  Demux/14 -> BusCreator/14  "TCU GearboxIn0 Clutch Trq_out"
  Demux/13 -> BusCreator/13  "TCU GearboxIn0 Clutch Trq_in"
  Demux/12 -> BusCreator/12  "TCU GearboxIn0 Clutch rotv_out_trg"
  Demux/11 -> BusCreator/11  "TCU GearboxIn0 Clutch rotv_out"
  Demux/10 -> BusCreator/10  "TCU GearboxIn0 Clutch rotv_in"
  Demux/9 -> BusCreator/9  "TCU GearboxIn0 Trq_out_trg"
  Demux/8 -> BusCreator/8  "TCU GearboxIn0 Trq_out"
  Demux/7 -> BusCreator/7  "TCU GearboxIn0 Trq_in"
  Demux/6 -> BusCreator/6  "TCU GearboxIn0 rotv_out"
  Demux/5 -> BusCreator/5  "TCU GearboxIn0 rotv_in_trg"
  Demux/4 -> BusCreator/4  "TCU GearboxIn0 rotv_in"
  Demux/3 -> BusCreator/3  "TCU GearboxIn0 i"
  Demux/2 -> BusCreator/2  "TCU GearboxIn0 GearNo_dis"
  Demux/1 -> BusCreator/1  "TCU GearboxIn0 GearNo"
  BusCreator/1 -> Out/1
  In/1 -> Demux/1

== system PTTransmCU/CarMaker/IPG Vehicle/PowerTrain/TCU Example/PTTransmCU_In/CreateBus TCU GearboxIn1 ==
  In : Inport
  BusCreator : BusCreator  Inputs=23
  Demux : Demux  Outputs=23
      settings: DisplayOption=none
  Out : Outport  VectorParamsAs1DForOutWhenUnconnected=off
  wires:
  Demux/23 -> BusCreator/23  "TCU GearboxIn1 Clutch_dis i_TrqIn2Out"
  Demux/22 -> BusCreator/22  "TCU GearboxIn1 Clutch_dis Trq_out_trg"
  Demux/21 -> BusCreator/21  "TCU GearboxIn1 Clutch_dis Trq_out"
  Demux/20 -> BusCreator/20  "TCU GearboxIn1 Clutch_dis Trq_in"
  Demux/19 -> BusCreator/19  "TCU GearboxIn1 Clutch_dis rotv_out_trg"
  Demux/18 -> BusCreator/18  "TCU GearboxIn1 Clutch_dis rotv_out"
  Demux/17 -> BusCreator/17  "TCU GearboxIn1 Clutch_dis rotv_in"
  Demux/16 -> BusCreator/16  "TCU GearboxIn1 Clutch i_TrqIn2Out"
  Demux/15 -> BusCreator/15  "TCU GearboxIn1 Clutch Trq_out_trg"
  Demux/14 -> BusCreator/14  "TCU GearboxIn1 Clutch Trq_out"
  Demux/13 -> BusCreator/13  "TCU GearboxIn1 Clutch Trq_in"
  Demux/12 -> BusCreator/12  "TCU GearboxIn1 Clutch rotv_out_trg"
  Demux/11 -> BusCreator/11  "TCU GearboxIn1 Clutch rotv_out"
  Demux/10 -> BusCreator/10  "TCU GearboxIn1 Clutch rotv_in"
  Demux/9 -> BusCreator/9  "TCU GearboxIn1 Trq_out_trg"
  Demux/8 -> BusCreator/8  "TCU GearboxIn1 Trq_out"
  Demux/7 -> BusCreator/7  "TCU GearboxIn1 Trq_in"
  Demux/6 -> BusCreator/6  "TCU GearboxIn1 rotv_out"
  Demux/5 -> BusCreator/5  "TCU GearboxIn1 rotv_in_trg"
  Demux/4 -> BusCreator/4  "TCU GearboxIn1 rotv_in"
  Demux/3 -> BusCreator/3  "TCU GearboxIn1 i"
  Demux/2 -> BusCreator/2  "TCU GearboxIn1 GearNo_dis"
  Demux/1 -> BusCreator/1  "TCU GearboxIn1 GearNo"
  BusCreator/1 -> Out/1
  In/1 -> Demux/1

== system PTTransmCU/CarMaker/IPG Vehicle/PowerTrain/TCU Example/PTTransmCU_In/CreateBus TCU GearboxIn10 ==
  In : Inport
  BusCreator : BusCreator  Inputs=23
  Demux : Demux  Outputs=23
      settings: DisplayOption=none
  Out : Outport  VectorParamsAs1DForOutWhenUnconnected=off
  wires:
  Demux/23 -> BusCreator/23  "TCU GearboxIn10 Clutch_dis i_TrqIn2Out"
  Demux/22 -> BusCreator/22  "TCU GearboxIn10 Clutch_dis Trq_out_trg"
  Demux/21 -> BusCreator/21  "TCU GearboxIn10 Clutch_dis Trq_out"
  Demux/20 -> BusCreator/20  "TCU GearboxIn10 Clutch_dis Trq_in"
  Demux/19 -> BusCreator/19  "TCU GearboxIn10 Clutch_dis rotv_out_trg"
  Demux/18 -> BusCreator/18  "TCU GearboxIn10 Clutch_dis rotv_out"
  Demux/17 -> BusCreator/17  "TCU GearboxIn10 Clutch_dis rotv_in"
  Demux/16 -> BusCreator/16  "TCU GearboxIn10 Clutch i_TrqIn2Out"
  Demux/15 -> BusCreator/15  "TCU GearboxIn10 Clutch Trq_out_trg"
  Demux/14 -> BusCreator/14  "TCU GearboxIn10 Clutch Trq_out"
  Demux/13 -> BusCreator/13  "TCU GearboxIn10 Clutch Trq_in"
  Demux/12 -> BusCreator/12  "TCU GearboxIn10 Clutch rotv_out_trg"
  Demux/11 -> BusCreator/11  "TCU GearboxIn10 Clutch rotv_out"
  Demux/10 -> BusCreator/10  "TCU GearboxIn10 Clutch rotv_in"
  Demux/9 -> BusCreator/9  "TCU GearboxIn10 Trq_out_trg"
  Demux/8 -> BusCreator/8  "TCU GearboxIn10 Trq_out"
  Demux/7 -> BusCreator/7  "TCU GearboxIn10 Trq_in"
  Demux/6 -> BusCreator/6  "TCU GearboxIn10 rotv_out"
  Demux/5 -> BusCreator/5  "TCU GearboxIn10 rotv_in_trg"
  Demux/4 -> BusCreator/4  "TCU GearboxIn10 rotv_in"
  Demux/3 -> BusCreator/3  "TCU GearboxIn10 i"
  Demux/2 -> BusCreator/2  "TCU GearboxIn10 GearNo_dis"
  Demux/1 -> BusCreator/1  "TCU GearboxIn10 GearNo"
  BusCreator/1 -> Out/1
  In/1 -> Demux/1

== system PTTransmCU/CarMaker/IPG Vehicle/PowerTrain/TCU Example/PTTransmCU_In/CreateBus TCU GearboxIn11 ==
  In : Inport
  BusCreator : BusCreator  Inputs=23
  Demux : Demux  Outputs=23
      settings: DisplayOption=none
  Out : Outport  VectorParamsAs1DForOutWhenUnconnected=off
  wires:
  Demux/23 -> BusCreator/23  "TCU GearboxIn11 Clutch_dis i_TrqIn2Out"
  Demux/22 -> BusCreator/22  "TCU GearboxIn11 Clutch_dis Trq_out_trg"
  Demux/21 -> BusCreator/21  "TCU GearboxIn11 Clutch_dis Trq_out"
  Demux/20 -> BusCreator/20  "TCU GearboxIn11 Clutch_dis Trq_in"
  Demux/19 -> BusCreator/19  "TCU GearboxIn11 Clutch_dis rotv_out_trg"
  Demux/18 -> BusCreator/18  "TCU GearboxIn11 Clutch_dis rotv_out"
  Demux/17 -> BusCreator/17  "TCU GearboxIn11 Clutch_dis rotv_in"
  Demux/16 -> BusCreator/16  "TCU GearboxIn11 Clutch i_TrqIn2Out"
  Demux/15 -> BusCreator/15  "TCU GearboxIn11 Clutch Trq_out_trg"
  Demux/14 -> BusCreator/14  "TCU GearboxIn11 Clutch Trq_out"
  Demux/13 -> BusCreator/13  "TCU GearboxIn11 Clutch Trq_in"
  Demux/12 -> BusCreator/12  "TCU GearboxIn11 Clutch rotv_out_trg"
  Demux/11 -> BusCreator/11  "TCU GearboxIn11 Clutch rotv_out"
  Demux/10 -> BusCreator/10  "TCU GearboxIn11 Clutch rotv_in"
  Demux/9 -> BusCreator/9  "TCU GearboxIn11 Trq_out_trg"
  Demux/8 -> BusCreator/8  "TCU GearboxIn11 Trq_out"
  Demux/7 -> BusCreator/7  "TCU GearboxIn11 Trq_in"
  Demux/6 -> BusCreator/6  "TCU GearboxIn11 rotv_out"
  Demux/5 -> BusCreator/5  "TCU GearboxIn11 rotv_in_trg"
  Demux/4 -> BusCreator/4  "TCU GearboxIn11 rotv_in"
  Demux/3 -> BusCreator/3  "TCU GearboxIn11 i"
  Demux/2 -> BusCreator/2  "TCU GearboxIn11 GearNo_dis"
  Demux/1 -> BusCreator/1  "TCU GearboxIn11 GearNo"
  BusCreator/1 -> Out/1
  In/1 -> Demux/1

== system PTTransmCU/CarMaker/IPG Vehicle/PowerTrain/TCU Example/PTTransmCU_In/CreateBus TCU GearboxIn2 ==
  In : Inport
  BusCreator : BusCreator  Inputs=23
  Demux : Demux  Outputs=23
      settings: DisplayOption=none
  Out : Outport  VectorParamsAs1DForOutWhenUnconnected=off
  wires:
  Demux/23 -> BusCreator/23  "TCU GearboxIn2 Clutch_dis i_TrqIn2Out"
  Demux/22 -> BusCreator/22  "TCU GearboxIn2 Clutch_dis Trq_out_trg"
  Demux/21 -> BusCreator/21  "TCU GearboxIn2 Clutch_dis Trq_out"
  Demux/20 -> BusCreator/20  "TCU GearboxIn2 Clutch_dis Trq_in"
  Demux/19 -> BusCreator/19  "TCU GearboxIn2 Clutch_dis rotv_out_trg"
  Demux/18 -> BusCreator/18  "TCU GearboxIn2 Clutch_dis rotv_out"
  Demux/17 -> BusCreator/17  "TCU GearboxIn2 Clutch_dis rotv_in"
  Demux/16 -> BusCreator/16  "TCU GearboxIn2 Clutch i_TrqIn2Out"
  Demux/15 -> BusCreator/15  "TCU GearboxIn2 Clutch Trq_out_trg"
  Demux/14 -> BusCreator/14  "TCU GearboxIn2 Clutch Trq_out"
  Demux/13 -> BusCreator/13  "TCU GearboxIn2 Clutch Trq_in"
  Demux/12 -> BusCreator/12  "TCU GearboxIn2 Clutch rotv_out_trg"
  Demux/11 -> BusCreator/11  "TCU GearboxIn2 Clutch rotv_out"
  Demux/10 -> BusCreator/10  "TCU GearboxIn2 Clutch rotv_in"
  Demux/9 -> BusCreator/9  "TCU GearboxIn2 Trq_out_trg"
  Demux/8 -> BusCreator/8  "TCU GearboxIn2 Trq_out"
  Demux/7 -> BusCreator/7  "TCU GearboxIn2 Trq_in"
  Demux/6 -> BusCreator/6  "TCU GearboxIn2 rotv_out"
  Demux/5 -> BusCreator/5  "TCU GearboxIn2 rotv_in_trg"
  Demux/4 -> BusCreator/4  "TCU GearboxIn2 rotv_in"
  Demux/3 -> BusCreator/3  "TCU GearboxIn2 i"
  Demux/2 -> BusCreator/2  "TCU GearboxIn2 GearNo_dis"
  Demux/1 -> BusCreator/1  "TCU GearboxIn2 GearNo"
  BusCreator/1 -> Out/1
  In/1 -> Demux/1

== system PTTransmCU/CarMaker/IPG Vehicle/PowerTrain/TCU Example/PTTransmCU_In/CreateBus TCU GearboxIn3 ==
  In : Inport
  BusCreator : BusCreator  Inputs=23
  Demux : Demux  Outputs=23
      settings: DisplayOption=none
  Out : Outport  VectorParamsAs1DForOutWhenUnconnected=off
  wires:
  Demux/23 -> BusCreator/23  "TCU GearboxIn3 Clutch_dis i_TrqIn2Out"
  Demux/22 -> BusCreator/22  "TCU GearboxIn3 Clutch_dis Trq_out_trg"
  Demux/21 -> BusCreator/21  "TCU GearboxIn3 Clutch_dis Trq_out"
  Demux/20 -> BusCreator/20  "TCU GearboxIn3 Clutch_dis Trq_in"
  Demux/19 -> BusCreator/19  "TCU GearboxIn3 Clutch_dis rotv_out_trg"
  Demux/18 -> BusCreator/18  "TCU GearboxIn3 Clutch_dis rotv_out"
  Demux/17 -> BusCreator/17  "TCU GearboxIn3 Clutch_dis rotv_in"
  Demux/16 -> BusCreator/16  "TCU GearboxIn3 Clutch i_TrqIn2Out"
  Demux/15 -> BusCreator/15  "TCU GearboxIn3 Clutch Trq_out_trg"
  Demux/14 -> BusCreator/14  "TCU GearboxIn3 Clutch Trq_out"
  Demux/13 -> BusCreator/13  "TCU GearboxIn3 Clutch Trq_in"
  Demux/12 -> BusCreator/12  "TCU GearboxIn3 Clutch rotv_out_trg"
  Demux/11 -> BusCreator/11  "TCU GearboxIn3 Clutch rotv_out"
  Demux/10 -> BusCreator/10  "TCU GearboxIn3 Clutch rotv_in"
  Demux/9 -> BusCreator/9  "TCU GearboxIn3 Trq_out_trg"
  Demux/8 -> BusCreator/8  "TCU GearboxIn3 Trq_out"
  Demux/7 -> BusCreator/7  "TCU GearboxIn3 Trq_in"
  Demux/6 -> BusCreator/6  "TCU GearboxIn3 rotv_out"
  Demux/5 -> BusCreator/5  "TCU GearboxIn3 rotv_in_trg"
  Demux/4 -> BusCreator/4  "TCU GearboxIn3 rotv_in"
  Demux/3 -> BusCreator/3  "TCU GearboxIn3 i"
  Demux/2 -> BusCreator/2  "TCU GearboxIn3 GearNo_dis"
  Demux/1 -> BusCreator/1  "TCU GearboxIn3 GearNo"
  BusCreator/1 -> Out/1
  In/1 -> Demux/1

== system PTTransmCU/CarMaker/IPG Vehicle/PowerTrain/TCU Example/PTTransmCU_In/CreateBus TCU GearboxIn4 ==
  In : Inport
  BusCreator : BusCreator  Inputs=23
  Demux : Demux  Outputs=23
      settings: DisplayOption=none
  Out : Outport  VectorParamsAs1DForOutWhenUnconnected=off
  wires:
  Demux/23 -> BusCreator/23  "TCU GearboxIn4 Clutch_dis i_TrqIn2Out"
  Demux/22 -> BusCreator/22  "TCU GearboxIn4 Clutch_dis Trq_out_trg"
  Demux/21 -> BusCreator/21  "TCU GearboxIn4 Clutch_dis Trq_out"
  Demux/20 -> BusCreator/20  "TCU GearboxIn4 Clutch_dis Trq_in"
  Demux/19 -> BusCreator/19  "TCU GearboxIn4 Clutch_dis rotv_out_trg"
  Demux/18 -> BusCreator/18  "TCU GearboxIn4 Clutch_dis rotv_out"
  Demux/17 -> BusCreator/17  "TCU GearboxIn4 Clutch_dis rotv_in"
  Demux/16 -> BusCreator/16  "TCU GearboxIn4 Clutch i_TrqIn2Out"
  Demux/15 -> BusCreator/15  "TCU GearboxIn4 Clutch Trq_out_trg"
  Demux/14 -> BusCreator/14  "TCU GearboxIn4 Clutch Trq_out"
  Demux/13 -> BusCreator/13  "TCU GearboxIn4 Clutch Trq_in"
  Demux/12 -> BusCreator/12  "TCU GearboxIn4 Clutch rotv_out_trg"
  Demux/11 -> BusCreator/11  "TCU GearboxIn4 Clutch rotv_out"
  Demux/10 -> BusCreator/10  "TCU GearboxIn4 Clutch rotv_in"
  Demux/9 -> BusCreator/9  "TCU GearboxIn4 Trq_out_trg"
  Demux/8 -> BusCreator/8  "TCU GearboxIn4 Trq_out"
  Demux/7 -> BusCreator/7  "TCU GearboxIn4 Trq_in"
  Demux/6 -> BusCreator/6  "TCU GearboxIn4 rotv_out"
  Demux/5 -> BusCreator/5  "TCU GearboxIn4 rotv_in_trg"
  Demux/4 -> BusCreator/4  "TCU GearboxIn4 rotv_in"
  Demux/3 -> BusCreator/3  "TCU GearboxIn4 i"
  Demux/2 -> BusCreator/2  "TCU GearboxIn4 GearNo_dis"
  Demux/1 -> BusCreator/1  "TCU GearboxIn4 GearNo"
  BusCreator/1 -> Out/1
  In/1 -> Demux/1

== system PTTransmCU/CarMaker/IPG Vehicle/PowerTrain/TCU Example/PTTransmCU_In/CreateBus TCU GearboxIn5 ==
  In : Inport
  BusCreator : BusCreator  Inputs=23
  Demux : Demux  Outputs=23
      settings: DisplayOption=none
  Out : Outport  VectorParamsAs1DForOutWhenUnconnected=off
  wires:
  Demux/23 -> BusCreator/23  "TCU GearboxIn5 Clutch_dis i_TrqIn2Out"
  Demux/22 -> BusCreator/22  "TCU GearboxIn5 Clutch_dis Trq_out_trg"
  Demux/21 -> BusCreator/21  "TCU GearboxIn5 Clutch_dis Trq_out"
  Demux/20 -> BusCreator/20  "TCU GearboxIn5 Clutch_dis Trq_in"
  Demux/19 -> BusCreator/19  "TCU GearboxIn5 Clutch_dis rotv_out_trg"
  Demux/18 -> BusCreator/18  "TCU GearboxIn5 Clutch_dis rotv_out"
  Demux/17 -> BusCreator/17  "TCU GearboxIn5 Clutch_dis rotv_in"
  Demux/16 -> BusCreator/16  "TCU GearboxIn5 Clutch i_TrqIn2Out"
  Demux/15 -> BusCreator/15  "TCU GearboxIn5 Clutch Trq_out_trg"
  Demux/14 -> BusCreator/14  "TCU GearboxIn5 Clutch Trq_out"
  Demux/13 -> BusCreator/13  "TCU GearboxIn5 Clutch Trq_in"
  Demux/12 -> BusCreator/12  "TCU GearboxIn5 Clutch rotv_out_trg"
  Demux/11 -> BusCreator/11  "TCU GearboxIn5 Clutch rotv_out"
  Demux/10 -> BusCreator/10  "TCU GearboxIn5 Clutch rotv_in"
  Demux/9 -> BusCreator/9  "TCU GearboxIn5 Trq_out_trg"
  Demux/8 -> BusCreator/8  "TCU GearboxIn5 Trq_out"
  Demux/7 -> BusCreator/7  "TCU GearboxIn5 Trq_in"
  Demux/6 -> BusCreator/6  "TCU GearboxIn5 rotv_out"
  Demux/5 -> BusCreator/5  "TCU GearboxIn5 rotv_in_trg"
  Demux/4 -> BusCreator/4  "TCU GearboxIn5 rotv_in"
  Demux/3 -> BusCreator/3  "TCU GearboxIn5 i"
  Demux/2 -> BusCreator/2  "TCU GearboxIn5 GearNo_dis"
  Demux/1 -> BusCreator/1  "TCU GearboxIn5 GearNo"
  BusCreator/1 -> Out/1
  In/1 -> Demux/1

== system PTTransmCU/CarMaker/IPG Vehicle/PowerTrain/TCU Example/PTTransmCU_In/CreateBus TCU GearboxIn6 ==
  In : Inport
  BusCreator : BusCreator  Inputs=23
  Demux : Demux  Outputs=23
      settings: DisplayOption=none
  Out : Outport  VectorParamsAs1DForOutWhenUnconnected=off
  wires:
  Demux/23 -> BusCreator/23  "TCU GearboxIn6 Clutch_dis i_TrqIn2Out"
  Demux/22 -> BusCreator/22  "TCU GearboxIn6 Clutch_dis Trq_out_trg"
  Demux/21 -> BusCreator/21  "TCU GearboxIn6 Clutch_dis Trq_out"
  Demux/20 -> BusCreator/20  "TCU GearboxIn6 Clutch_dis Trq_in"
  Demux/19 -> BusCreator/19  "TCU GearboxIn6 Clutch_dis rotv_out_trg"
  Demux/18 -> BusCreator/18  "TCU GearboxIn6 Clutch_dis rotv_out"
  Demux/17 -> BusCreator/17  "TCU GearboxIn6 Clutch_dis rotv_in"
  Demux/16 -> BusCreator/16  "TCU GearboxIn6 Clutch i_TrqIn2Out"
  Demux/15 -> BusCreator/15  "TCU GearboxIn6 Clutch Trq_out_trg"
  Demux/14 -> BusCreator/14  "TCU GearboxIn6 Clutch Trq_out"
  Demux/13 -> BusCreator/13  "TCU GearboxIn6 Clutch Trq_in"
  Demux/12 -> BusCreator/12  "TCU GearboxIn6 Clutch rotv_out_trg"
  Demux/11 -> BusCreator/11  "TCU GearboxIn6 Clutch rotv_out"
  Demux/10 -> BusCreator/10  "TCU GearboxIn6 Clutch rotv_in"
  Demux/9 -> BusCreator/9  "TCU GearboxIn6 Trq_out_trg"
  Demux/8 -> BusCreator/8  "TCU GearboxIn6 Trq_out"
  Demux/7 -> BusCreator/7  "TCU GearboxIn6 Trq_in"
  Demux/6 -> BusCreator/6  "TCU GearboxIn6 rotv_out"
  Demux/5 -> BusCreator/5  "TCU GearboxIn6 rotv_in_trg"
  Demux/4 -> BusCreator/4  "TCU GearboxIn6 rotv_in"
  Demux/3 -> BusCreator/3  "TCU GearboxIn6 i"
  Demux/2 -> BusCreator/2  "TCU GearboxIn6 GearNo_dis"
  Demux/1 -> BusCreator/1  "TCU GearboxIn6 GearNo"
  BusCreator/1 -> Out/1
  In/1 -> Demux/1

== system PTTransmCU/CarMaker/IPG Vehicle/PowerTrain/TCU Example/PTTransmCU_In/CreateBus TCU GearboxIn7 ==
  In : Inport
  BusCreator : BusCreator  Inputs=23
  Demux : Demux  Outputs=23
      settings: DisplayOption=none
  Out : Outport  VectorParamsAs1DForOutWhenUnconnected=off
  wires:
  Demux/23 -> BusCreator/23  "TCU GearboxIn7 Clutch_dis i_TrqIn2Out"
  Demux/22 -> BusCreator/22  "TCU GearboxIn7 Clutch_dis Trq_out_trg"
  Demux/21 -> BusCreator/21  "TCU GearboxIn7 Clutch_dis Trq_out"
  Demux/20 -> BusCreator/20  "TCU GearboxIn7 Clutch_dis Trq_in"
  Demux/19 -> BusCreator/19  "TCU GearboxIn7 Clutch_dis rotv_out_trg"
  Demux/18 -> BusCreator/18  "TCU GearboxIn7 Clutch_dis rotv_out"
  Demux/17 -> BusCreator/17  "TCU GearboxIn7 Clutch_dis rotv_in"
  Demux/16 -> BusCreator/16  "TCU GearboxIn7 Clutch i_TrqIn2Out"
  Demux/15 -> BusCreator/15  "TCU GearboxIn7 Clutch Trq_out_trg"
  Demux/14 -> BusCreator/14  "TCU GearboxIn7 Clutch Trq_out"
  Demux/13 -> BusCreator/13  "TCU GearboxIn7 Clutch Trq_in"
  Demux/12 -> BusCreator/12  "TCU GearboxIn7 Clutch rotv_out_trg"
  Demux/11 -> BusCreator/11  "TCU GearboxIn7 Clutch rotv_out"
  Demux/10 -> BusCreator/10  "TCU GearboxIn7 Clutch rotv_in"
  Demux/9 -> BusCreator/9  "TCU GearboxIn7 Trq_out_trg"
  Demux/8 -> BusCreator/8  "TCU GearboxIn7 Trq_out"
  Demux/7 -> BusCreator/7  "TCU GearboxIn7 Trq_in"
  Demux/6 -> BusCreator/6  "TCU GearboxIn7 rotv_out"
  Demux/5 -> BusCreator/5  "TCU GearboxIn7 rotv_in_trg"
  Demux/4 -> BusCreator/4  "TCU GearboxIn7 rotv_in"
  Demux/3 -> BusCreator/3  "TCU GearboxIn7 i"
  Demux/2 -> BusCreator/2  "TCU GearboxIn7 GearNo_dis"
  Demux/1 -> BusCreator/1  "TCU GearboxIn7 GearNo"
  BusCreator/1 -> Out/1
  In/1 -> Demux/1
